simulink model "rvs_testing"  (R2016a)
settings: Solver=FixedStepDiscrete  StartTime=0.0  StopTime=10.0  RelTol=1e-3
libraries: rvs x13
settings Model: Creator=Arthur  LastModifiedBy=aeagr
settings DataIOCC: LimitDataPoints=on  SaveFormat=Array
settings DebuggingCC: SolverPrmCheckMsg=warning
settings HardwareCC: ProdBitPerPointer=32  ProdLargestAtomicFloat=None  ProdIntDivRoundTo=Undefined  ProdEndianess=Unspecified  ProdWordSize=32  ProdHWDeviceType=32-bit Generic
settings ModelReferenceCC: PropagateSignalLabelsOutOfModel=off
settings ConfigComp: CovModelRefEnable=Off  CovSFcnEnable=off

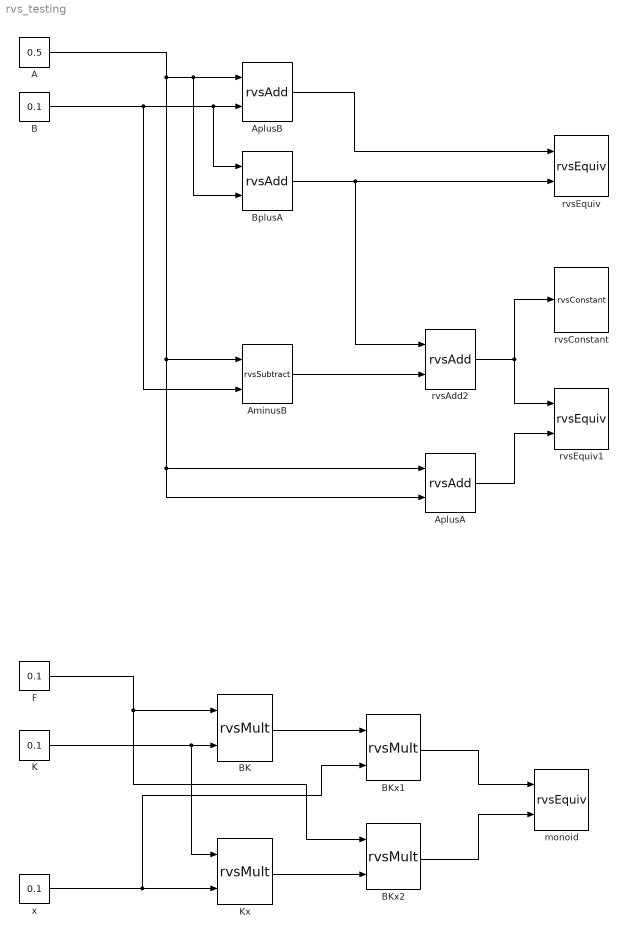
== system rvs_testing ==
  A : Constant  Value=0.5
  AminusB : rvs/rvsSubtract
  AplusA : rvs/rvsAdd
  AplusB : rvs/rvsAdd
  B : Constant  Value=0.1
  BK : rvs/rvsMult
  BKx1 : rvs/rvsMult
  BKx2 : rvs/rvsMult
  BplusA : rvs/rvsAdd
  F : Constant  Value=0.1
  K : Constant  Value=0.1
  Kx : rvs/rvsMult
  monoid : rvs/rvsEquiv  tol=1e-9
  rvsAdd2 : rvs/rvsAdd
  rvsConstant : rvs/rvsConstant
  rvsEquiv : rvs/rvsEquiv  tol=1e-9
  rvsEquiv1 : rvs/rvsEquiv  tol=1e-9
  x : Constant  Value=0.1
  wires:
  B/1 -> AminusB/2, BplusA/1, AplusB/2
  AplusB/1 -> rvsEquiv/1
  AminusB/1 -> rvsAdd2/2
  BplusA/1 -> rvsAdd2/1, rvsEquiv/2
  rvsAdd2/1 -> rvsConstant/1, rvsEquiv1/1
  AplusA/1 -> rvsEquiv1/2
  A/1 -> AplusA/2, AplusA/1, AminusB/1, BplusA/2, AplusB/1
  K/1 -> Kx/1, BK/2
  BK/1 -> BKx1/1
  x/1 -> Kx/2, BKx1/2
  Kx/1 -> BKx2/2
  BKx1/1 -> monoid/1
  BKx2/1 -> monoid/2
  F/1 -> BKx2/1, BK/1
